simulink model "C_framewiseincremental_vs_framewiseglobal"  (R2017a)
settings: Solver=ode45  StartTime=0.0  StopTime=200  FixedStep=0.05  RelTol=1e-3  EnableMultiTasking=on
values from neighbouring files (symbols this model uses):
  B = [1 0.5 -0.5 -1 0 0.5 ; 0 0 0 0 2 0 ; -0.05 -0.02 0.02 0.05 0 2 ; -1 -1 -1 -1 -2 0]    [A_runSimulation.m]    (also in C_runSimulation.m; D_runSimulation.m; E_runSimulation.m; F_runSimulation.m)
  gain_four = rand()*2    [A_runSimulation.m]    (also in C_runSimulation.m = 0; D_runSimulation.m; E_runSimulation.m = 0; F_runSimulation.m = 0)
  gain_one = rand()*2    [A_runSimulation.m]    (also in C_runSimulation.m = 0; D_runSimulation.m; E_runSimulation.m = 0; F_runSimulation.m = 0)
  gain_three = rand()*2    [A_runSimulation.m]    (also in C_runSimulation.m = 0; D_runSimulation.m; E_runSimulation.m = 0; F_runSimulation.m = 0)
  gain_two = rand()*2    [A_runSimulation.m]    (also in C_runSimulation.m = 0; D_runSimulation.m; E_runSimulation.m = 0; F_runSimulation.m = 0)
  reduction_type = 1    [A_runSimulation.m]    (also in C_runSimulation.m = 2; D_runSimulation.m; E_runSimulation.m = 2)
  seed_four = k + 30    [A_runSimulation.m]    (also in C_runSimulation.m; D_runSimulation.m; E_runSimulation.m; F_runSimulation.m)
  seed_one = k    [A_runSimulation.m]    (also in C_runSimulation.m; D_runSimulation.m; E_runSimulation.m; F_runSimulation.m)
  seed_three = k + 20    [A_runSimulation.m]    (also in C_runSimulation.m; D_runSimulation.m; E_runSimulation.m; F_runSimulation.m)
  seed_two = k + 10    [A_runSimulation.m]    (also in C_runSimulation.m; D_runSimulation.m; E_runSimulation.m; F_runSimulation.m)
  signal_gain = j    [A_runSimulation.m]    (also in C_runSimulation.m; D_runSimulation.m; E_runSimulation.m = 0.3; F_runSimulation.m)
  simulate_envelope = 1    [A_runSimulation.m]    (also in C_runSimulation.m = 0; D_runSimulation.m; E_runSimulation.m = 0)
  u_lim = [[-0.5 -0.5 -0.5 -0.5 -0.5 -0.5]' [0.5 0.5 0.5 0.5 0.5 0.5]']    [A_runSimulation.m]    (also in C_runSimulation.m; D_runSimulation.m; E_runSimulation.m; F_runSimulation.m)
  udot_lim = [[2 2 2 2 2 2]']    [A_runSimulation.m]    (also in C_runSimulation.m; D_runSimulation.m; E_runSimulation.m; F_runSimulation.m)
  W = eye(6)    [A_runSimulation.m]    (also in C_runSimulation.m; D_runSimulation.m; E_runSimulation.m; F_runSimulation.m)
libraries: dspsrcs4 x8
settings Model: Creator=markvoskuijl  LastModifiedBy=Luca
settings DataIOCC: LimitDataPoints=on  SaveFormat=Array  SignalLoggingSaveFormat=ModelDataLogs
settings OptimizationCC: ExpressionDepthLimit=2147483647  LifeSpan=inf
settings DebuggingCC: UnderspecifiedInitializationDetection=Classic  MergeDetectMultiDrivingBlocksExec=none  SolverPrmCheckMsg=warning  FcnCallInpInsideContextMsg=warning  StateNameClashWarn=warning  SFUnexpectedBacktrackingDiag=warning  SFNoUnconditionalDefaultTransitionDiag=warning  SFExecutionAtInitializationDiag=none
settings HardwareCC: ProdBitPerPointer=32  ProdBitPerSizeT=32  ProdBitPerPtrDiffT=32  ProdLargestAtomicFloat=None  ProdIntDivRoundTo=Undefined  ProdEndianess=Unspecified  ProdWordSize=32  ProdHWDeviceType=32-bit Generic
settings ModelReferenceCC: PropagateSignalLabelsOutOfModel=off
settings GRTTargetCC: TargetLangStandard=C89/C90 (ANSI)  GeneratePreprocessorConditionals=Disable all  CombineOutputUpdateFcns=off  GRTInterface=on
settings ConfigComp: CovMetricSettings=dw  CovHtmlReporting=on  CovSaveCumulativeToWorkspaceVar=on  CovSaveSingleToWorkspaceVar=on  CovExternalEMLEnable=off

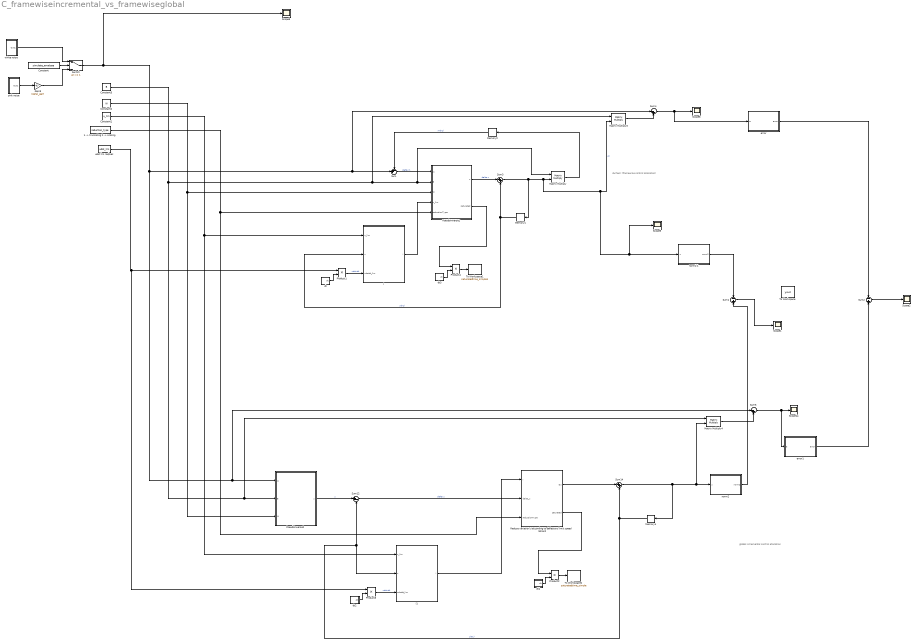
== system C_framewiseincremental_vs_framewiseglobal ==
  note: global incremental control allocation
  note: durham
      | (framewise control allocation)
  "1 -> truncating 2 -> scaling" : Constant  Value=reduction_type
  Constant : Constant  Value=simulate_envelope
  Constant1 : Constant  Value=u_lim
  Constant2 : Constant  Value=W
  Constant3 : Constant  Value=B
  Gain3 : Gain  Gain=signal_gain
  I : MATLAB Function  TreatAsAtomicUnit=on
  I1 : MATLAB Function  TreatAsAtomicUnit=on
  Matrix Multiply : Product  Multiplication=Matrix(*)
  Matrix Multiply3 : Product  Multiplication=Matrix(*)
  Matrix Multiply4 : Product  Multiplication=Matrix(*)
  Memory1 : Memory
  Memory2 : Memory
  Memory4 : Memory
  Product{1..4} (4 alike) : Product
  Pseudoinverse1 : MATLAB Function  TreatAsAtomicUnit=on
  Pseudoinverse2 : MATLAB Function  TreatAsAtomicUnit=on
  Reduce variation u according to deflectors limit speed ratios2 : MATLAB Function  TreatAsAtomicUnit=on
  Scope{1..3,5..6,14} (6 alike) : Scope
  Sum : Sum  Inputs=-+|
  Sum1 : Sum  Inputs=-|+
  Sum12 : Sum  Inputs=|+-
  Sum14 : Sum  Inputs=|++
  Sum2 : Sum  Inputs=-|+
  Sum3 : Sum  Inputs=|++
  Sum4 : Sum  Inputs=|-+
  Sum5 : Sum  Inputs=|-+
  Switch : Switch  Threshold=1
  To Workspace : ToWorkspace  VariableName=yout  SampleTime=-1
      settings: Save2DSignal=2-D array (concatenate along first dimension)
  To Workspace1 : ToWorkspace  VariableName=saturatedtime_simple1  SampleTime=-1
      settings: Save2DSignal=2-D array (concatenate along first dimension)
  To Workspace2 : ToWorkspace  VariableName=saturatedtime_simple  SampleTime=-1
      settings: Save2DSignal=2-D array (concatenate along first dimension)
  dt : Subsystem
  dt1 : Subsystem
  dt2 : Subsystem
  dt3 : Subsystem
  error : MATLAB Function  TreatAsAtomicUnit=on
  error1 : MATLAB Function  TreatAsAtomicUnit=on
  "norm2 " : MATLAB Function  TreatAsAtomicUnit=on
  norm2 1 : MATLAB Function  TreatAsAtomicUnit=on
  pink noise : Subsystem
  udot lim rad/sec : Constant  Value=udot_lim
  white noise : Subsystem
  wires:
  Sum/1 -> Pseudoinverse1/1(m)  "delta m"
  Matrix Multiply/1 -> Memory2/1
  I/1(I) -> Pseudoinverse1/4(u_lim)
  Pseudoinverse1/1(u) -> Sum3/1  "delta u"
  Product1/1 -> I/3(udotdt_lim)  "udot dt"
  dt/1(dt) -> Product1/2
  Memory1/1 -> I/2(u), Sum3/2  "u(t-1)"
  Memory2/1 -> Sum/1  "m(t-1)"
  Matrix Multiply3/1 -> Sum4/2
  Sum4/1 -> error/1(e), Scope6/1
  Sum3/1 -> Memory1/1, Scope5/1, norm2 1/1(u), Matrix Multiply3/2, Matrix Multiply/2  "ut"
  Constant2/1 -> Pseudoinverse2/3(W), Pseudoinverse1/3(W)
  Pseudoinverse2/1(u) -> Sum12/1  "u"
  Reduce variation u according to deflectors limit speed ratios2/1(Du) -> Sum14/1
  Memory4/1 -> Sum14/2, Sum12/2, I1/2(u)  "u(t-1)"
  Sum12/1 -> Reduce variation u according to deflectors limit speed ratios2/2(delta_u)  "delta u"
  I1/1(I) -> Reduce variation u according to deflectors limit speed ratios2/1(I)
  dt2/1(dt) -> Product3/2
  udot lim rad/sec/1 -> Product3/1, Product1/1
  Product3/1 -> I1/3(udotdt_lim)  "udot dt"
  Constant1/1 -> I1/1(u_lim), I/1(u_lim)
  "1 -> truncating 2 -> scaling"/1 -> Reduce variation u according to deflectors limit speed ratios2/3(reductionType), Pseudoinverse1/5(reductionType)
  Sum14/1 -> "norm2 "/1(u), Matrix Multiply4/2, Memory4/1
  Sum5/1 -> error1/1(e), Scope14/1
  Constant3/1 -> Matrix Multiply4/1, Pseudoinverse2/2(B), Matrix Multiply3/1, Matrix Multiply/1, Pseudoinverse1/2(B)
  Matrix Multiply4/1 -> Sum5/2
  "norm2 "/1(norm2) -> Sum1/2
  norm2 1/1(norm2) -> Sum1/1
  Sum1/1 -> Scope1/1
  error1/1(error) -> Sum2/2
  error/1(error) -> Sum2/1
  Sum2/1 -> Scope2/1
  Switch/1 -> Scope3/1, Sum5/1, Pseudoinverse2/1(m), Sum4/1, Sum/2
  white noise/1(Out1) -> Switch/1
  Gain3/1 -> Switch/3
  Constant/1 -> Switch/2
  pink noise/1(Out1) -> Gain3/1
  Product4/1 -> To Workspace1/1
  dt3/1(dt) -> Product4/2
  Pseudoinverse1/2(saturated) -> Product4/1
  Product2/1 -> To Workspace2/1
  dt1/1(dt) -> Product2/2
  Reduce variation u according to deflectors limit speed ratios2/2(saturated) -> Product2/1

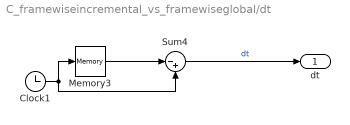
== system C_framewiseincremental_vs_framewiseglobal/dt ==
  Clock1 : Clock
  Memory3 : Memory
  Sum4 : Sum  Inputs=|-+
  dt : Outport
  wires:
  Clock1/1 -> Sum4/2, Memory3/1
  Memory3/1 -> Sum4/1
  Sum4/1 -> dt/1  "dt"

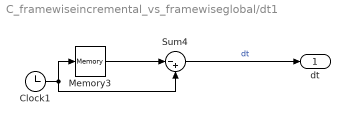
== system C_framewiseincremental_vs_framewiseglobal/dt1 ==
  Clock1 : Clock
  Memory3 : Memory
  Sum4 : Sum  Inputs=|-+
  dt : Outport
  wires:
  Clock1/1 -> Sum4/2, Memory3/1
  Memory3/1 -> Sum4/1
  Sum4/1 -> dt/1  "dt"

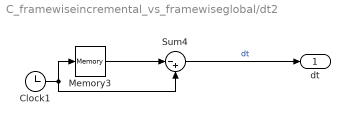
== system C_framewiseincremental_vs_framewiseglobal/dt2 ==
  Clock1 : Clock
  Memory3 : Memory
  Sum4 : Sum  Inputs=|-+
  dt : Outport
  wires:
  Clock1/1 -> Sum4/2, Memory3/1
  Memory3/1 -> Sum4/1
  Sum4/1 -> dt/1  "dt"

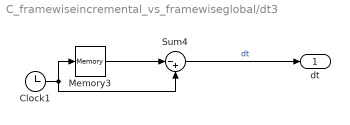
== system C_framewiseincremental_vs_framewiseglobal/dt3 ==
  Clock1 : Clock
  Memory3 : Memory
  Sum4 : Sum  Inputs=|-+
  dt : Outport
  wires:
  Clock1/1 -> Sum4/2, Memory3/1
  Memory3/1 -> Sum4/1
  Sum4/1 -> dt/1  "dt"

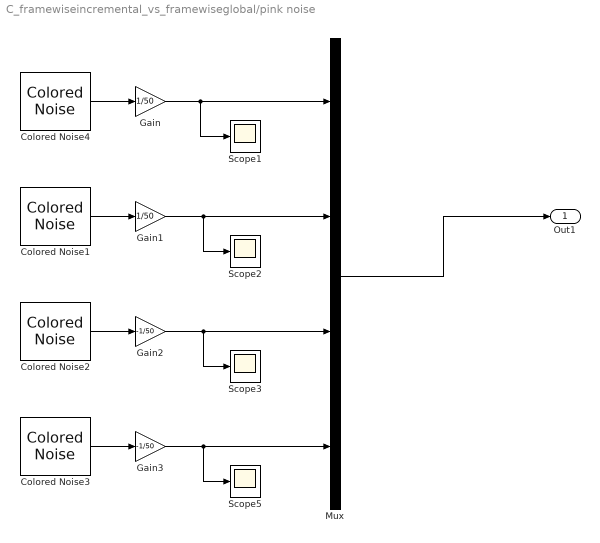
== system C_framewiseincremental_vs_framewiseglobal/pink noise ==
  Colored Noise1 : dspsrcs4/Colored Noise  Color=custom  InverseFrequencyPower=2  NumChannels=1  OutputDataType=single  SamplesPerFrame=1  SampleTime=0.1  RandomStream=mt19937ar with seed  Seed=seed_two  SimulateUsing=Interpreted execution
      settings: SourceProductName=DSP System Toolbox  SourceProductBaseCode=DS
  Colored Noise2 : dspsrcs4/Colored Noise  Color=custom  InverseFrequencyPower=2  NumChannels=1  OutputDataType=single  SamplesPerFrame=1  SampleTime=0.1  RandomStream=mt19937ar with seed  Seed=seed_three  SimulateUsing=Interpreted execution
      settings: SourceProductName=DSP System Toolbox  SourceProductBaseCode=DS
  Colored Noise3 : dspsrcs4/Colored Noise  Color=custom  InverseFrequencyPower=2  NumChannels=1  OutputDataType=single  SamplesPerFrame=1  SampleTime=0.1  RandomStream=mt19937ar with seed  Seed=seed_four  SimulateUsing=Interpreted execution
      settings: SourceProductName=DSP System Toolbox  SourceProductBaseCode=DS
  Colored Noise4 : dspsrcs4/Colored Noise  Color=custom  InverseFrequencyPower=2  NumChannels=1  OutputDataType=single  SamplesPerFrame=1  SampleTime=0.1  RandomStream=mt19937ar with seed  Seed=seed_one  SimulateUsing=Interpreted execution
      settings: SourceProductName=DSP System Toolbox  SourceProductBaseCode=DS
  Gain : Gain  Gain=1/50
  Gain1 : Gain  Gain=1/50
  Gain2 : Gain  Gain=-1/50
  Gain3 : Gain  Gain=-1/50
  Mux : Mux
  Scope{1..3,5} (4 alike) : Scope
  Out1 : Outport
  wires:
  Colored Noise4/1 -> Gain/1
  Colored Noise1/1 -> Gain1/1
  Colored Noise2/1 -> Gain2/1
  Gain/1 -> Scope1/1, Mux/1
  Gain1/1 -> Scope2/1, Mux/2
  Gain2/1 -> Scope3/1, Mux/3
  Mux/1 -> Out1/1
  Gain3/1 -> Mux/4, Scope5/1
  Colored Noise3/1 -> Gain3/1

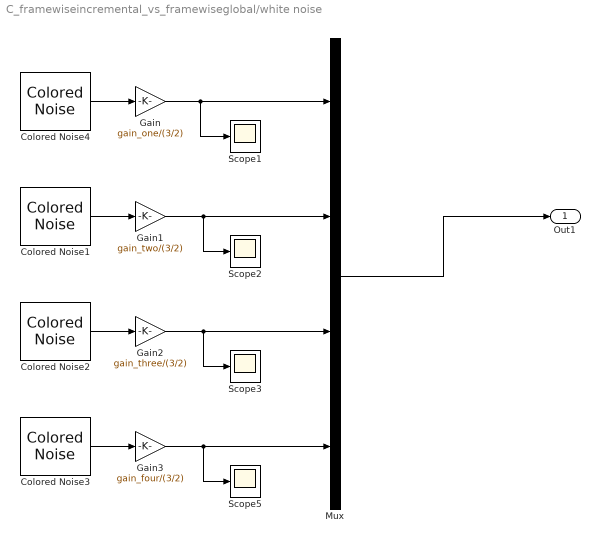
== system C_framewiseincremental_vs_framewiseglobal/white noise ==
  Colored Noise1 : dspsrcs4/Colored Noise  Color=white  InverseFrequencyPower=2  NumChannels=1  OutputDataType=single  SamplesPerFrame=1  SampleTime=0.1  RandomStream=mt19937ar with seed  Seed=seed_two  SimulateUsing=Interpreted execution
      settings: SourceProductName=DSP System Toolbox  SourceProductBaseCode=DS
  Colored Noise2 : dspsrcs4/Colored Noise  Color=white  InverseFrequencyPower=2  NumChannels=1  OutputDataType=single  SamplesPerFrame=1  SampleTime=0.1  RandomStream=mt19937ar with seed  Seed=seed_three  SimulateUsing=Interpreted execution
      settings: SourceProductName=DSP System Toolbox  SourceProductBaseCode=DS
  Colored Noise3 : dspsrcs4/Colored Noise  Color=white  InverseFrequencyPower=2  NumChannels=1  OutputDataType=single  SamplesPerFrame=1  SampleTime=0.1  RandomStream=mt19937ar with seed  Seed=seed_four  SimulateUsing=Interpreted execution
      settings: SourceProductName=DSP System Toolbox  SourceProductBaseCode=DS
  Colored Noise4 : dspsrcs4/Colored Noise  Color=white  InverseFrequencyPower=2  NumChannels=1  OutputDataType=single  SamplesPerFrame=1  SampleTime=0.1  RandomStream=mt19937ar with seed  Seed=seed_one  SimulateUsing=Interpreted execution
      settings: SourceProductName=DSP System Toolbox  SourceProductBaseCode=DS
  Gain : Gain  Gain=gain_one/(3/2)
  Gain1 : Gain  Gain=gain_two/(3/2)
  Gain2 : Gain  Gain=gain_three/(3/2)
  Gain3 : Gain  Gain=gain_four/(3/2)
  Mux : Mux
  Scope{1..3,5} (4 alike) : Scope
  Out1 : Outport
  wires:
  Colored Noise4/1 -> Gain/1
  Colored Noise1/1 -> Gain1/1
  Colored Noise2/1 -> Gain2/1
  Gain/1 -> Scope1/1, Mux/1
  Gain1/1 -> Scope2/1, Mux/2
  Gain2/1 -> Scope3/1, Mux/3
  Mux/1 -> Out1/1
  Gain3/1 -> Mux/4, Scope5/1
  Colored Noise3/1 -> Gain3/1

== matlab function C_framewiseincremental_vs_framewiseglobal/Pseudoinverse1 ==
  data: m input; u output; B input; W input; u_lim input; reductionType input; saturated output
function [u , saturated] = Pseudoinverse(m, B, W, u_lim, reductionType)
coder.varsize('u_index', 'Br', 'Wr', 'u_sat');

%check if the matrices are correct
    if not(isequal(size(u_lim,1),size(B,2),size(W,1),size(W,2))...
       && isequal(length(m),size(B,1)))
        error ('input matrix dimensions do not match')
    end
    
%assign to every equation an index    
    u_index = [1:length(u_lim)].';
    
%check the type of system and then compute the pseudoinverse 1st step
    order = size(B,2)-size(B,1);

    if order > 0 %over-determined, solution that minimizes the 2norm
        u = inv(W)*B'*inv(B*inv(W)*B')*m;
    elseif order < 0 %under-determined, solution that minimizes the error
        u = inv(B'*B)*B'*m;   
    else %order = 0, sqared thus invertiBrle
        u = inv(B)*m;
    end

%deifne u_sat vector
    u_sat = zeros(length(u),1);
    
    saturated = 0;
    
%check if the first iteration solution is correct then return    
    if not(any(u < u_lim(:,1))||any(u > u_lim(:,2)))  
        return
    end
    
    
%The software continues only if the solution has to be reduced
    saturated = 1;
    
%reduce their value
    switch reductionType
        case 1 %truncation
            %takes note of which one are out of their bounds
                u_sat(u < u_lim(:,1)) = 1;
                u_sat(u > u_lim(:,2)) = 1;
                
            %trucate
                u = min(u, u_lim(:,2));
                u = max(u, u_lim(:,1));

        case 2 %scaling solution -> direction preserving
            %reduce
                a = zeros(length(u),1);

                for i = 1:length(u)
                    if u(i)>0
                       a(i) = abs(u(i)/u_lim(i,2));
                    elseif u(i)<0
                       a(i) = abs(u(i)/u_lim(i,1));
                    else
                       a(i) = 0; 
                    end          
                end
                a_max = max(a);
                u = u/a_max;
            
            %takes note of which one are out of their bounds
                u_sat(u == u_lim(:,2)) = 1;
                u_sat(u == u_lim(:,1)) = 1;
            
    end
    
return
    
end

== matlab function C_framewiseincremental_vs_framewiseglobal/norm2  ==
  data: u input; norm2 output
function norm2 = norm2(u)

    norm2 = sum(u.^2);

end

== matlab function C_framewiseincremental_vs_framewiseglobal/norm2 1 ==
  data: u input; norm2 output
function norm2 = norm2(u)

    norm2 = sum(u.^2);

end

== matlab function C_framewiseincremental_vs_framewiseglobal/I ==
  data: u_lim input; u input; udotdt_lim input; I output
function I = computeIntersection(u_lim, u, udotdt_lim)
%check if the matrices are correct
    if not(isequal(size(u_lim,1),size(udotdt_lim,1), size(u,1)))
        error ('input matrix dimensions do not match')
    end

%declare space of intersection
    I = zeros(length(u_lim),2);
    
    I(:,1) = -min(udotdt_lim, abs(u_lim(:,1)-u));
    I(:,2) = min(+udotdt_lim, abs(u_lim(:,2)-u));
    
end

== matlab function C_framewiseincremental_vs_framewiseglobal/Pseudoinverse2 ==
  data: m input; u output; B input; W input
function u = PseudoinverseSimple(m, B, W)
coder.varsize('u_index', 'Br', 'Wr', 'u_sat');

%check if the matrices are correct
    if not(isequal(size(B,2),size(W,1),size(W,2))...
       && isequal(length(m),size(B,1)))
        error ('input matrix dimensions do not match')
    end
   
%check the type of system and then compute the pseudoinverse 1st step
    order = size(B,2)-size(B,1);

    if order > 0 %over-determined, solution that minimizes the 2norm
        u = inv(W)*B'*inv(B*inv(W)*B')*m;
    elseif order < 0 %under-determined, solution that minimizes the error
        u = inv(B'*B)*B'*m;   
    else %order = 0, sqared thus invertiBrle
        u = inv(B)*m;
    end
 
end

== matlab function C_framewiseincremental_vs_framewiseglobal/I1 ==
  data: u_lim input; u input; udotdt_lim input; I output
function I = computeIntersection(u_lim, u, udotdt_lim)
%check if the matrices are correct
    if not(isequal(size(u_lim,1),size(udotdt_lim,1), size(u,1)))
        error ('input matrix dimensions do not match')
    end

%declare space of intersection
    I = zeros(length(u_lim),2);
    
    I(:,1) = -min(udotdt_lim, abs(u_lim(:,1)-u));
    I(:,2) = min(+udotdt_lim, abs(u_lim(:,2)-u));
    
end

== matlab function C_framewiseincremental_vs_framewiseglobal/error ==
  data: e input; error output
function error = error(e)

    error = sum(abs(e));

end

== matlab function C_framewiseincremental_vs_framewiseglobal/error1 ==
  data: e input; error output
function error = error(e)

    error = sum(abs(e));

end

== matlab function C_framewiseincremental_vs_framewiseglobal/Reduce variation u according to deflectors limit speed ratios2 ==
  data: I input; Du output; delta_u input; reductionType input; saturated output
function [Du , saturated] = Reduce(I, delta_u, reductionType)

%check if the matrices are correct
    if not(isequal(size(delta_u,1),size(I,1)))
        error ('input matrix dimensions do not match')
    end

%first aproximation    
    Du = delta_u; 
    
    saturated = 0;
    
%if some control effectors are saturated, reduce them
    if (any(delta_u < I(:,1))||any(delta_u > I(:,2)))
        saturated = 1;
        
        switch reductionType
            case 1 %truncation
                    Du = min(delta_u, I(:,2));
                    Du = max(Du, I(:,1));

            case 2 %scaling solution -> direction preserving
                %reduce
                    a = zeros(length(delta_u),1);

                    for i = 1:length(delta_u)
                        if delta_u(i)>0
                           a(i) = abs(delta_u(i)/I(i,2));
                        elseif delta_u(i)<0
                           a(i) = abs(delta_u(i)/I(i,1));
                        else
                           a(i) = 0; 
                        end          
                    end
                    a_max = max(a);
                    Du = delta_u/a_max;
        end
    end

end
